simulink model "RLFactoryEnforceCrash6Opponents"  (R2020a)
settings: Solver=VariableStepAuto  StartTime=0.0  StopTime=60  RelTol=1e-3
undefined symbols (not defined in the file): BLOCKEDTIMER, EPS, getRandomSafeCoord, GoalRange, MAXVELOA, MAXVELOB, MAXVELOC, MAXVELOD, MAXVELOE, MAXVELOF, rl, RLStartX, RLStartY, SAFETYDISTANCEA, SAFETYDISTANCEB, SAFETYDISTANCEC, SAFETYDISTANCED, SAFETYDISTANCEE, SAFETYDISTANCEF, THRESHOLDA, THRESHOLDB, THRESHOLDC, THRESHOLDD, THRESHOLDE, THRESHOLDF, TSA, TSB, TSC, TSD, TSE, TSF, TSRL
libraries: rllib x1
(part 1 of 3)
settings Model: Creator=julius  LastModifiedBy=julius

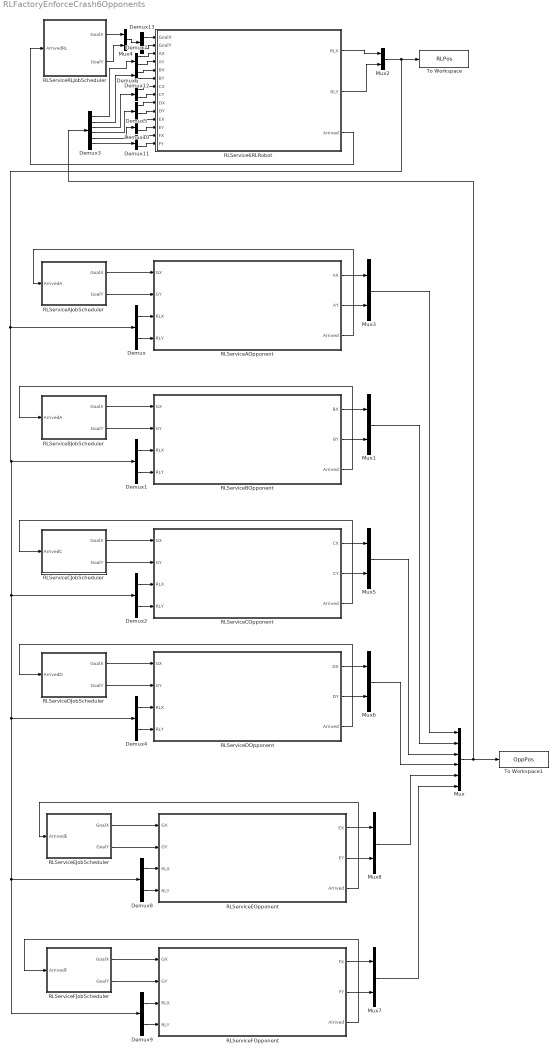
== system RLFactoryEnforceCrash6Opponents ==
  Demux{,1..2,4..13} (13 alike) : Demux  Outputs=2
  Demux3 : Demux  Outputs=6
  Mux : Mux  Inputs=6
  Mux{1..8} (8 alike) : Mux  Inputs=2
  RLService6RLRobot : Subsystem
  RLServiceAJobScheduler : Subsystem
  RLServiceAOpponent : Subsystem
  RLServiceBJobScheduler : Subsystem
  RLServiceBOpponent : Subsystem
  RLServiceCJobScheduler : Subsystem
  RLServiceCOpponent : Subsystem
  RLServiceDJobScheduler : Subsystem
  RLServiceDOpponent : Subsystem
  RLServiceEJobScheduler : Subsystem
  RLServiceEOpponent : Subsystem
  RLServiceFJobScheduler : Subsystem
  RLServiceFOpponent : Subsystem
  RLServiceRLJobScheduler : Subsystem
  To Workspace : ToWorkspace  VariableName=RLPos  SampleTime=TSRL
  To Workspace1 : ToWorkspace  VariableName=OppPos  SampleTime=TSRL
  wires:
  RLServiceAJobScheduler/1(GoalX) -> RLServiceAOpponent/1(GX)
  RLServiceAJobScheduler/2(GoalY) -> RLServiceAOpponent/2(GY)
  RLServiceAOpponent/3(Arrived) -> RLServiceAJobScheduler/1(ArrivedA)
  Demux/1 -> RLServiceAOpponent/3(RLX)
  Demux/2 -> RLServiceAOpponent/4(RLY)
  RLServiceBJobScheduler/1(GoalX) -> RLServiceBOpponent/1(GX)
  RLServiceBJobScheduler/2(GoalY) -> RLServiceBOpponent/2(GY)
  Demux1/1 -> RLServiceBOpponent/3(RLX)
  Demux1/2 -> RLServiceBOpponent/4(RLY)
  RLServiceBOpponent/1(BX) -> Mux1/1
  RLServiceBOpponent/2(BY) -> Mux1/2
  RLServiceAOpponent/1(AX) -> Mux3/1
  RLServiceAOpponent/2(AY) -> Mux3/2
  RLServiceBOpponent/3(Arrived) -> RLServiceBJobScheduler/1(ArrivedA)
  RLServiceRLJobScheduler/2(GoalY) -> Mux4/2
  RLServiceRLJobScheduler/1(GoalX) -> Mux4/1
  Mux4/1 -> Demux13/1
  Mux3/1 -> Mux/1
  Mux1/1 -> Mux/2
  Mux/1 -> Demux3/1, To Workspace1/1
  Demux3/1 -> Demux7/1
  Demux3/2 -> Demux12/1
  Demux13/1 -> RLService6RLRobot/1(GoalX)
  Demux13/2 -> RLService6RLRobot/2(GoalY)
  Demux7/1 -> RLService6RLRobot/3(AX)
  Demux7/2 -> RLService6RLRobot/4(AY)
  Demux12/1 -> RLService6RLRobot/5(BX)
  Demux12/2 -> RLService6RLRobot/6(BY)
  RLService6RLRobot/3(Arrived) -> RLServiceRLJobScheduler/1(ArrivedRL)
  RLService6RLRobot/1(RLX) -> Mux2/1
  RLService6RLRobot/2(RLY) -> Mux2/2
  RLServiceCJobScheduler/2(GoalY) -> RLServiceCOpponent/2(GY)
  Demux2/2 -> RLServiceCOpponent/4(RLY)
  RLServiceCOpponent/2(CY) -> Mux5/2
  RLServiceCJobScheduler/1(GoalX) -> RLServiceCOpponent/1(GX)
  RLServiceCOpponent/3(Arrived) -> RLServiceCJobScheduler/1(ArrivedC)
  RLServiceCOpponent/1(CX) -> Mux5/1
  Demux2/1 -> RLServiceCOpponent/3(RLX)
  RLServiceDJobScheduler/2(GoalY) -> RLServiceDOpponent/2(GY)
  Demux4/2 -> RLServiceDOpponent/4(RLY)
  RLServiceDOpponent/2(DY) -> Mux6/2
  RLServiceDJobScheduler/1(GoalX) -> RLServiceDOpponent/1(GX)
  RLServiceDOpponent/3(Arrived) -> RLServiceDJobScheduler/1(ArrivedD)
  RLServiceDOpponent/1(DX) -> Mux6/1
  Demux4/1 -> RLServiceDOpponent/3(RLX)
  Mux5/1 -> Mux/3
  Mux6/1 -> Mux/4
  Demux6/2 -> RLService6RLRobot/8(CY)
  Demux3/3 -> Demux6/1
  Demux6/1 -> RLService6RLRobot/7(CX)
  Demux8/2 -> RLServiceEOpponent/4(RLY)
  RLServiceEOpponent/1(EX) -> Mux8/1
  RLServiceEJobScheduler/1(GoalX) -> RLServiceEOpponent/1(GX)
  RLServiceEOpponent/2(EY) -> Mux8/2
  Mux8/1 -> Mux/5
  Demux8/1 -> RLServiceEOpponent/3(RLX)
  Demux9/2 -> RLServiceFOpponent/4(RLY)
  RLServiceFOpponent/3(Arrived) -> RLServiceFJobScheduler/1(ArrivedF)
  RLServiceEOpponent/3(Arrived) -> RLServiceEJobScheduler/1(ArrivedE)
  RLServiceFOpponent/1(FX) -> Mux7/1
  RLServiceEJobScheduler/2(GoalY) -> RLServiceEOpponent/2(GY)
  RLServiceFJobScheduler/1(GoalX) -> RLServiceFOpponent/1(GX)
  Mux2/1 -> Demux8/1, Demux9/1, Demux4/1, Demux2/1, Demux1/1, Demux/1, To Workspace/1
  RLServiceFOpponent/2(FY) -> Mux7/2
  Mux7/1 -> Mux/6
  RLServiceFJobScheduler/2(GoalY) -> RLServiceFOpponent/2(GY)
  Demux9/1 -> RLServiceFOpponent/3(RLX)
  Demux5/1 -> RLService6RLRobot/9(DX)
  Demux5/2 -> RLService6RLRobot/10(DY)
  Demux3/4 -> Demux5/1
  Demux10/1 -> RLService6RLRobot/11(EX)
  Demux10/2 -> RLService6RLRobot/12(EY)
  Demux11/1 -> RLService6RLRobot/13(FX)
  Demux11/2 -> RLService6RLRobot/14(FY)
  Demux3/5 -> Demux10/1
  Demux3/6 -> Demux11/1

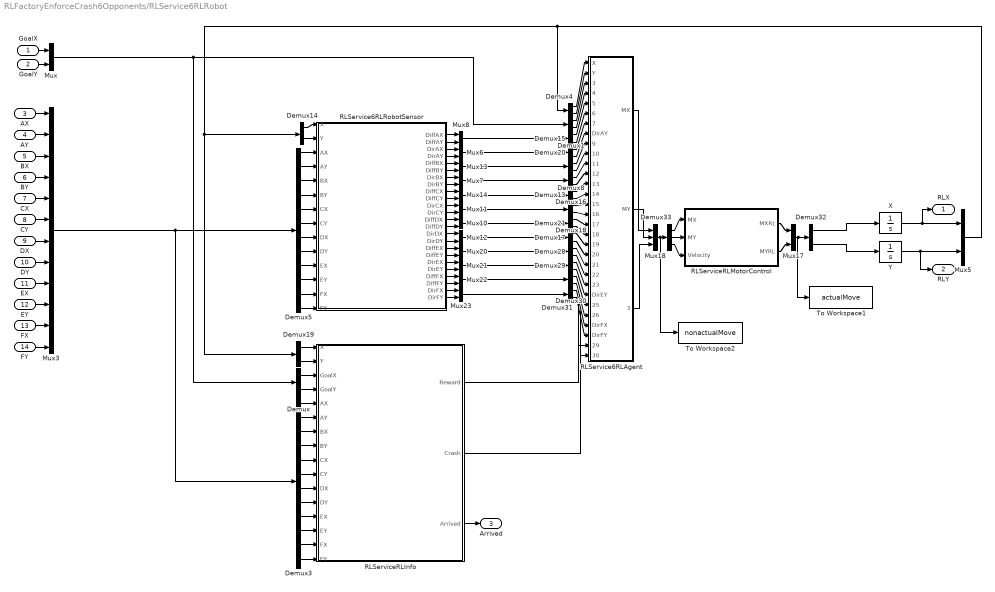
== system RLFactoryEnforceCrash6Opponents/RLService6RLRobot ==
  GoalX : Inport
  GoalY : Inport  Port=2
  AX : Inport  Port=3
  AY : Inport  Port=4
  BX : Inport  Port=5
  BY : Inport  Port=6
  CX : Inport  Port=7
  CY : Inport  Port=8
  DX : Inport  Port=9
  DY : Inport  Port=10
  EX : Inport  Port=11
  EY : Inport  Port=12
  FX : Inport  Port=13
  FY : Inport  Port=14
  Demux{,1,4,8,13..21,28..32} (18 alike) : Demux  Outputs=2
  Demux3 : Demux  Outputs=12
  Demux33 : Demux  Outputs=3
  Demux5 : Demux  Outputs=12
  Mux{,5..8,10..14,17,20..23} (15 alike) : Mux  Inputs=2
  Mux18 : Mux  Inputs=3
  Mux3 : Mux  Inputs=12
  RLService6RLAgent : Subsystem
  RLService6RLRobotSensor : Subsystem
  RLServiceRLInfo : Subsystem
  RLServiceRLMotorControl : Subsystem
  To Workspace1 : ToWorkspace  VariableName=actualMove  SampleTime=-1
  To Workspace2 : ToWorkspace  VariableName=nonactualMove  SampleTime=-1
  X : Integrator  InitialCondition=RLStartX
  Y : Integrator  InitialCondition=RLStartY
  RLX : Outport
  RLY : Outport  Port=2
  Arrived : Outport  Port=3
  wires:
  AX/1 -> Mux3/1
  X/1 -> Mux5/1, RLX/1
  Mux13/1 -> Demux8/1
  Demux19/1 -> RLServiceRLInfo/1(X)
  Demux4/1 -> RLService6RLAgent/1(X)
  Demux4/2 -> RLService6RLAgent/2(Y)
  Demux15/1 -> RLService6RLAgent/5(DiffAX)
  GoalX/1 -> Mux/1
  Demux20/2 -> RLService6RLAgent/8(DirAY)
  Demux19/2 -> RLServiceRLInfo/2(Y)
  Demux1/2 -> RLService6RLAgent/4(GoalY)
  Demux16/1 -> RLService6RLAgent/11(DirBX)
  Demux15/2 -> RLService6RLAgent/6(DiffAY)
  Demux/2 -> RLServiceRLInfo/4(GoalY)
  Demux1/1 -> RLService6RLAgent/3(GoalX)
  Y/1 -> RLY/1, Mux5/2
  RLService6RLAgent/2(MY) -> Mux18/2
  Mux3/1 -> Demux5/1, Demux3/1
  Demux20/1 -> RLService6RLAgent/7(DirAX)
  Demux8/1 -> RLService6RLAgent/9(DiffBX)
  BY/1 -> Mux3/4
  GoalY/1 -> Mux/2
  Mux5/1 -> Demux14/1, Demux19/1, Demux4/1
  Mux6/1 -> Demux20/1
  Demux/1 -> RLServiceRLInfo/3(GoalX)
  RLService6RLAgent/1(MX) -> Mux18/1
  Mux7/1 -> Demux16/1
  BX/1 -> Mux3/3
  Demux16/2 -> RLService6RLAgent/12(DirBY)
  AY/1 -> Mux3/2
  Demux8/2 -> RLService6RLAgent/10(DiffBY)
  Mux8/1 -> Demux15/1
  RLService6RLAgent/3(Velocity) -> Mux18/3
  CX/1 -> Mux3/5
  CY/1 -> Mux3/6
  DX/1 -> Mux3/7
  DY/1 -> Mux3/8
  Demux13/1 -> RLService6RLAgent/13(DiffCX)
  Demux18/2 -> RLService6RLAgent/16(DirCY)
  Demux13/2 -> RLService6RLAgent/14(DiffCY)
  Demux21/2 -> RLService6RLAgent/18(DiffDY)
  Demux17/1 -> RLService6RLAgent/19(DirDX)
  Demux17/2 -> RLService6RLAgent/20(DirDY)
  Demux18/1 -> RLService6RLAgent/15(DirCX)
  Demux21/1 -> RLService6RLAgent/17(DiffDX)
  Mux14/1 -> Demux13/1
  Mux11/1 -> Demux18/1
  Mux10/1 -> Demux21/1
  Mux12/1 -> Demux17/1
  FX/1 -> Mux3/11
  EY/1 -> Mux3/10
  EX/1 -> Mux3/9
  FY/1 -> Mux3/12
  Demux14/1 -> RLService6RLRobotSensor/1(X)
  Demux14/2 -> RLService6RLRobotSensor/2(Y)
  RLService6RLRobotSensor/1(DiffAX) -> Mux8/1
  RLService6RLRobotSensor/2(DiffAY) -> Mux8/2
  Mux/1 -> Demux1/1, Demux/1
  RLService6RLRobotSensor/3(DirAX) -> Mux6/1
  RLService6RLRobotSensor/4(DirAY) -> Mux6/2
  RLService6RLRobotSensor/5(DiffBX) -> Mux13/1
  RLService6RLRobotSensor/6(DiffBY) -> Mux13/2
  RLService6RLRobotSensor/7(DirBX) -> Mux7/1
  RLService6RLRobotSensor/8(DirBY) -> Mux7/2
  RLService6RLRobotSensor/9(DiffCX) -> Mux14/1
  RLService6RLRobotSensor/10(DiffCY) -> Mux14/2
  RLService6RLRobotSensor/11(DirCX) -> Mux11/1
  RLService6RLRobotSensor/12(DirCY) -> Mux11/2
  RLService6RLRobotSensor/13(DiffDX) -> Mux10/1
  RLService6RLRobotSensor/14(DiffDY) -> Mux10/2
  RLService6RLRobotSensor/15(DirDX) -> Mux12/1
  RLService6RLRobotSensor/16(DirDY) -> Mux12/2
  RLService6RLRobotSensor/17(DiffEX) -> Mux20/1
  RLService6RLRobotSensor/18(DiffEY) -> Mux20/2
  Demux28/1 -> RLService6RLAgent/21(DiffEX)
  Demux28/2 -> RLService6RLAgent/22(DiffEY)
  Mux20/1 -> Demux28/1
  Demux29/2 -> RLService6RLAgent/24(DirEY)
  Demux29/1 -> RLService6RLAgent/23(DirEX)
  RLService6RLRobotSensor/19(DirEX) -> Mux21/1
  RLService6RLRobotSensor/20(DirEY) -> Mux21/2
  Mux21/1 -> Demux29/1
  RLService6RLRobotSensor/21(DiffFX) -> Mux22/1
  RLService6RLRobotSensor/22(DiffFY) -> Mux22/2
  Demux30/1 -> RLService6RLAgent/25(DiffFX)
  Demux30/2 -> RLService6RLAgent/26(DiffFY)
  Mux22/1 -> Demux30/1
  RLService6RLRobotSensor/23(DirFX) -> Mux23/1
  RLService6RLRobotSensor/24(DirFY) -> Mux23/2
  Mux23/1 -> Demux31/1
  Demux31/1 -> RLService6RLAgent/27(DirFX)
  Demux31/2 -> RLService6RLAgent/28(DirFY)
  RLServiceRLMotorControl/1(MXRL) -> Mux17/1
  RLServiceRLMotorControl/2(MYRL) -> Mux17/2
  Mux17/1 -> To Workspace1/1, Demux32/1
  Demux32/1 -> X/1
  Demux32/2 -> Y/1
  Demux33/1 -> RLServiceRLMotorControl/1(MX)
  Demux33/2 -> RLServiceRLMotorControl/2(MY)
  Demux33/3 -> RLServiceRLMotorControl/3(Velocity)
  Mux18/1 -> Demux33/1, To Workspace2/1
  RLServiceRLInfo/3(Arrived) -> Arrived/1
  Demux3/1 -> RLServiceRLInfo/5(AX)
  Demux3/2 -> RLServiceRLInfo/6(AY)
  Demux3/3 -> RLServiceRLInfo/7(BX)
  Demux3/4 -> RLServiceRLInfo/8(BY)
  Demux3/5 -> RLServiceRLInfo/9(CX)
  Demux3/6 -> RLServiceRLInfo/10(CY)
  Demux3/7 -> RLServiceRLInfo/11(DX)
  Demux3/8 -> RLServiceRLInfo/12(DY)
  Demux3/9 -> RLServiceRLInfo/13(EX)
  Demux3/10 -> RLServiceRLInfo/14(EY)
  Demux3/11 -> RLServiceRLInfo/15(FX)
  Demux3/12 -> RLServiceRLInfo/16(FY)
  RLServiceRLInfo/1(Reward) -> RLService6RLAgent/29(Reward)
  RLServiceRLInfo/2(Crash) -> RLService6RLAgent/30(IsDone)
  Demux5/2 -> RLService6RLRobotSensor/4(AY)
  Demux5/3 -> RLService6RLRobotSensor/5(BX)
  Demux5/4 -> RLService6RLRobotSensor/6(BY)
  Demux5/5 -> RLService6RLRobotSensor/7(CX)
  Demux5/6 -> RLService6RLRobotSensor/8(CY)
  Demux5/7 -> RLService6RLRobotSensor/9(DX)
  Demux5/8 -> RLService6RLRobotSensor/10(DY)
  Demux5/9 -> RLService6RLRobotSensor/11(EX)
  Demux5/10 -> RLService6RLRobotSensor/12(EY)
  Demux5/11 -> RLService6RLRobotSensor/13(FX)
  Demux5/12 -> RLService6RLRobotSensor/14(FY)
  Demux5/1 -> RLService6RLRobotSensor/3(AX)

== system RLFactoryEnforceCrash6Opponents/RLServiceAJobScheduler ==
  ArrivedA : Inport
  Constant1 : Constant  Value=[[randi([-GoalRange,GoalRange],1),randi([-GoalRange,GoalRange],1)];[randi([-GoalRange,GoalRange],1),randi([-GoalRange,GoalRange],1)]]
  JobScheduler2 : MATLABSystem  System=JobScheduler  SimulateUsing=Interpreted execution
      mask Type: JobScheduler
      mask Display:
      | disp('JobScheduler');
      | port_label('input',1,'workstations');
      | port_label('input',2,'done');
      | port_label('output',1,'currentGoalX');
      | port_label('output',2,'currentGoalY');
  GoalX : Outport
  GoalY : Outport  Port=2
  wires:
  Constant1/1 -> JobScheduler2/1
  JobScheduler2/2 -> GoalY/1
  ArrivedA/1 -> JobScheduler2/2
  JobScheduler2/1 -> GoalX/1

== system RLFactoryEnforceCrash6Opponents/RLServiceAOpponent ==
  GX : Inport
  GY : Inport  Port=2
  RLX : Inport  Port=3
  RLY : Inport  Port=4
  Constant1 : Constant  Value=MAXVELOA
  Constant2 : Constant  Value=TSA
  Constant3 : Constant  Value=THRESHOLDA
  Demux : Demux  Outputs=6
  Demux1 : Demux  Outputs=2
  Demux11 : Demux  Outputs=3
  Demux2 : Demux  Outputs=2
  Mux : Mux  Inputs=2
  Mux2 : Mux  Inputs=3
  Mux9 : Mux  Inputs=6
  RLServiceAOpponentController : Subsystem
  X : Integrator  InitialCondition=getRandomSafeCoord(RLStartX,SAFETYDISTANCEA,EPS)
  Y : Integrator  InitialCondition=getRandomSafeCoord(RLStartY,SAFETYDISTANCEA,EPS)
  ZOA : ZeroOrderHold  SampleTime=TSA
  AX : Outport
  AY : Outport  Port=2
  Arrived : Outport  Port=3
  wires:
  RLServiceAOpponentController/1(Arrived) -> Arrived/1
  Demux/4 -> RLServiceAOpponentController/4(GoalY)
  Demux/6 -> RLServiceAOpponentController/6(RLY)
  X/1 -> Mux/1
  RLY/1 -> Mux9/6
  Demux/5 -> RLServiceAOpponentController/5(RLX)
  GY/1 -> Mux9/4
  Demux/1 -> RLServiceAOpponentController/1(X)
  Y/1 -> Mux/2
  Mux/1 -> Demux1/1, Demux2/1
  Mux9/1 -> ZOA/1
  Demux/3 -> RLServiceAOpponentController/3(GoalX)
  Demux/2 -> RLServiceAOpponentController/2(Y)
  RLX/1 -> Mux9/5
  ZOA/1 -> Demux/1
  GX/1 -> Mux9/3
  Mux2/1 -> Demux11/1
  Demux1/1 -> Mux9/1
  Demux1/2 -> Mux9/2
  Constant2/1 -> Mux2/2
  Constant1/1 -> Mux2/1
  Constant3/1 -> Mux2/3
  Demux2/1 -> AX/1
  Demux2/2 -> AY/1
  RLServiceAOpponentController/3(MY) -> Y/1
  RLServiceAOpponentController/2(MX) -> X/1
  Demux11/1 -> RLServiceAOpponentController/7(MaxVelo)
  Demux11/2 -> RLServiceAOpponentController/8(TS)
  Demux11/3 -> RLServiceAOpponentController/9(THRESHOLD)

== system RLFactoryEnforceCrash6Opponents/RLServiceBJobScheduler ==
  ArrivedA : Inport
  Constant1 : Constant  Value=[[randi([-GoalRange,GoalRange],1),randi([-GoalRange,GoalRange],1)];[randi([-GoalRange,GoalRange],1),randi([-GoalRange,GoalRange],1)]]
  JobScheduler2 : MATLABSystem  System=JobScheduler  SimulateUsing=Interpreted execution
      mask Type: JobScheduler
      mask Display:
      | disp('JobScheduler');
      | port_label('input',1,'workstations');
      | port_label('input',2,'done');
      | port_label('output',1,'currentGoalX');
      | port_label('output',2,'currentGoalY');
  GoalX : Outport
  GoalY : Outport  Port=2
  wires:
  Constant1/1 -> JobScheduler2/1
  JobScheduler2/2 -> GoalY/1
  ArrivedA/1 -> JobScheduler2/2
  JobScheduler2/1 -> GoalX/1

== system RLFactoryEnforceCrash6Opponents/RLServiceBOpponent ==
  GX : Inport
  GY : Inport  Port=2
  RLX : Inport  Port=3
  RLY : Inport  Port=4
  Constant1 : Constant  Value=MAXVELOB
  Constant2 : Constant  Value=TSB
  Constant3 : Constant  Value=THRESHOLDB
  Demux : Demux  Outputs=6
  Demux1 : Demux  Outputs=2
  Demux11 : Demux  Outputs=3
  Demux2 : Demux  Outputs=2
  Mux : Mux  Inputs=2
  Mux2 : Mux  Inputs=3
  Mux9 : Mux  Inputs=6
  RLServiceAOpponentController : Subsystem
  X : Integrator  InitialCondition=getRandomSafeCoord(RLStartX,SAFETYDISTANCEB,EPS)
  Y : Integrator  InitialCondition=getRandomSafeCoord(RLStartY,SAFETYDISTANCEB,EPS)
  ZOB : ZeroOrderHold  SampleTime=TSB
  BX : Outport
  BY : Outport  Port=2
  Arrived : Outport  Port=3
  wires:
  RLServiceAOpponentController/3(MY) -> Y/1
  RLX/1 -> Mux9/5
  Demux11/1 -> RLServiceAOpponentController/7(MaxVelo)
  Constant2/1 -> Mux2/2
  RLServiceAOpponentController/2(MX) -> X/1
  Mux9/1 -> ZOB/1
  Constant3/1 -> Mux2/3
  Demux1/2 -> Mux9/2
  Demux/1 -> RLServiceAOpponentController/1(X)
  GY/1 -> Mux9/4
  Demux/4 -> RLServiceAOpponentController/4(GoalY)
  RLServiceAOpponentController/1(Arrived) -> Arrived/1
  X/1 -> Mux/1
  Mux/1 -> Demux1/1, Demux2/1
  Demux/6 -> RLServiceAOpponentController/6(RLY)
  Demux/3 -> RLServiceAOpponentController/3(GoalX)
  Demux1/1 -> Mux9/1
  Demux11/2 -> RLServiceAOpponentController/8(TS)
  Demux2/1 -> BX/1
  RLY/1 -> Mux9/6
  Demux/2 -> RLServiceAOpponentController/2(Y)
  Demux11/3 -> RLServiceAOpponentController/9(THRESHOLD)
  ZOB/1 -> Demux/1
  Demux2/2 -> BY/1
  Mux2/1 -> Demux11/1
  Constant1/1 -> Mux2/1
  GX/1 -> Mux9/3
  Y/1 -> Mux/2
  Demux/5 -> RLServiceAOpponentController/5(RLX)

== system RLFactoryEnforceCrash6Opponents/RLServiceCJobScheduler ==
  ArrivedC : Inport
  Constant1 : Constant  Value=[[randi([-5,5],1),randi([-5,5],1)];[randi([-5,5],1),randi([-5,5],1)]]
  JobScheduler2 : MATLABSystem  System=JobScheduler  SimulateUsing=Interpreted execution
      mask Type: JobScheduler
      mask Display:
      | disp('JobScheduler');
      | port_label('input',1,'workstations');
      | port_label('input',2,'done');
      | port_label('output',1,'currentGoalX');
      | port_label('output',2,'currentGoalY');
  GoalX : Outport
  GoalY : Outport  Port=2
  wires:
  Constant1/1 -> JobScheduler2/1
  JobScheduler2/2 -> GoalY/1
  ArrivedC/1 -> JobScheduler2/2
  JobScheduler2/1 -> GoalX/1

== system RLFactoryEnforceCrash6Opponents/RLServiceCOpponent ==
  GX : Inport
  GY : Inport  Port=2
  RLX : Inport  Port=3
  RLY : Inport  Port=4
  Constant1 : Constant  Value=MAXVELOC
  Constant2 : Constant  Value=TSC
  Constant3 : Constant  Value=THRESHOLDC
  Demux : Demux  Outputs=6
  Demux1 : Demux  Outputs=2
  Demux11 : Demux  Outputs=3
  Demux2 : Demux  Outputs=2
  Mux : Mux  Inputs=2
  Mux2 : Mux  Inputs=3
  Mux9 : Mux  Inputs=6
  RLServiceAOpponentController : Subsystem
  X : Integrator  InitialCondition=getRandomSafeCoord(RLStartX,SAFETYDISTANCEC,EPS)
  Y : Integrator  InitialCondition=getRandomSafeCoord(RLStartY,SAFETYDISTANCEC,EPS)
  ZOC : ZeroOrderHold  SampleTime=TSC
  CX : Outport
  CY : Outport  Port=2
  Arrived : Outport  Port=3
  wires:
  RLServiceAOpponentController/3(MY) -> Y/1
  RLX/1 -> Mux9/5
  Demux11/1 -> RLServiceAOpponentController/7(MaxVelo)
  Constant2/1 -> Mux2/2
  RLServiceAOpponentController/2(MX) -> X/1
  Mux9/1 -> ZOC/1
  Constant3/1 -> Mux2/3
  Demux1/2 -> Mux9/2
  Demux/1 -> RLServiceAOpponentController/1(X)
  GY/1 -> Mux9/4
  Demux/4 -> RLServiceAOpponentController/4(GoalY)
  RLServiceAOpponentController/1(Arrived) -> Arrived/1
  X/1 -> Mux/1
  Mux/1 -> Demux1/1, Demux2/1
  Demux/6 -> RLServiceAOpponentController/6(RLY)
  Demux/3 -> RLServiceAOpponentController/3(GoalX)
  Demux1/1 -> Mux9/1
  Demux11/2 -> RLServiceAOpponentController/8(TS)
  Demux2/1 -> CX/1
  RLY/1 -> Mux9/6
  Demux/2 -> RLServiceAOpponentController/2(Y)
  Demux11/3 -> RLServiceAOpponentController/9(THRESHOLD)
  ZOC/1 -> Demux/1
  Demux2/2 -> CY/1
  Mux2/1 -> Demux11/1
  Constant1/1 -> Mux2/1
  GX/1 -> Mux9/3
  Y/1 -> Mux/2
  Demux/5 -> RLServiceAOpponentController/5(RLX)

== system RLFactoryEnforceCrash6Opponents/RLServiceDJobScheduler ==
  ArrivedD : Inport
  Constant1 : Constant  Value=[[randi([-GoalRange,GoalRange],1),randi([-GoalRange,GoalRange],1)];[randi([-GoalRange,GoalRange],1),randi([-GoalRange,GoalRange],1)]]
  JobScheduler2 : MATLABSystem  System=JobScheduler  SimulateUsing=Interpreted execution
      mask Type: JobScheduler
      mask Display:
      | disp('JobScheduler');
      | port_label('input',1,'workstations');
      | port_label('input',2,'done');
      | port_label('output',1,'currentGoalX');
      | port_label('output',2,'currentGoalY');
  GoalX : Outport
  GoalY : Outport  Port=2
  wires:
  Constant1/1 -> JobScheduler2/1
  JobScheduler2/2 -> GoalY/1
  ArrivedD/1 -> JobScheduler2/2
  JobScheduler2/1 -> GoalX/1

== system RLFactoryEnforceCrash6Opponents/RLServiceDOpponent ==
  GX : Inport
  GY : Inport  Port=2
  RLX : Inport  Port=3
  RLY : Inport  Port=4
  Constant1 : Constant  Value=MAXVELOD
  Constant2 : Constant  Value=TSD
  Constant3 : Constant  Value=THRESHOLDD
  Demux : Demux  Outputs=6
  Demux1 : Demux  Outputs=2
  Demux11 : Demux  Outputs=3
  Demux2 : Demux  Outputs=2
  Mux : Mux  Inputs=2
  Mux2 : Mux  Inputs=3
  Mux9 : Mux  Inputs=6
  RLServiceAOpponentController : Subsystem
  X : Integrator  InitialCondition=getRandomSafeCoord(RLStartX,SAFETYDISTANCED,EPS)
  Y : Integrator  InitialCondition=getRandomSafeCoord(RLStartY,SAFETYDISTANCED,EPS)
  ZOB : ZeroOrderHold  SampleTime=TSD
  DX : Outport
  DY : Outport  Port=2
  Arrived : Outport  Port=3
  wires:
  RLServiceAOpponentController/3(MY) -> Y/1
  RLX/1 -> Mux9/5
  Demux11/1 -> RLServiceAOpponentController/7(MaxVelo)
  Constant2/1 -> Mux2/2
  RLServiceAOpponentController/2(MX) -> X/1
  Mux9/1 -> ZOB/1
  Constant3/1 -> Mux2/3
  Demux1/2 -> Mux9/2
  Demux/1 -> RLServiceAOpponentController/1(X)
  GY/1 -> Mux9/4
  Demux/4 -> RLServiceAOpponentController/4(GoalY)
  RLServiceAOpponentController/1(Arrived) -> Arrived/1
  X/1 -> Mux/1
  Mux/1 -> Demux1/1, Demux2/1
  Demux/6 -> RLServiceAOpponentController/6(RLY)
  Demux/3 -> RLServiceAOpponentController/3(GoalX)
  Demux1/1 -> Mux9/1
  Demux11/2 -> RLServiceAOpponentController/8(TS)
  Demux2/1 -> DX/1
  RLY/1 -> Mux9/6
  Demux/2 -> RLServiceAOpponentController/2(Y)
  Demux11/3 -> RLServiceAOpponentController/9(THRESHOLD)
  ZOB/1 -> Demux/1
  Demux2/2 -> DY/1
  Mux2/1 -> Demux11/1
  Constant1/1 -> Mux2/1
  GX/1 -> Mux9/3
  Y/1 -> Mux/2
  Demux/5 -> RLServiceAOpponentController/5(RLX)

== system RLFactoryEnforceCrash6Opponents/RLServiceEJobScheduler ==
  ArrivedE : Inport
  Constant1 : Constant  Value=[[randi([-GoalRange,GoalRange],1),randi([-GoalRange,GoalRange],1)];[randi([-GoalRange,GoalRange],1),randi([-GoalRange,GoalRange],1)]]
  JobScheduler2 : MATLABSystem  System=JobScheduler  SimulateUsing=Interpreted execution
      mask Type: JobScheduler
      mask Display:
      | disp('JobScheduler');
      | port_label('input',1,'workstations');
      | port_label('input',2,'done');
      | port_label('output',1,'currentGoalX');
      | port_label('output',2,'currentGoalY');
  GoalX : Outport
  GoalY : Outport  Port=2
  wires:
  Constant1/1 -> JobScheduler2/1
  JobScheduler2/2 -> GoalY/1
  ArrivedE/1 -> JobScheduler2/2
  JobScheduler2/1 -> GoalX/1

== system RLFactoryEnforceCrash6Opponents/RLServiceEOpponent ==
  GX : Inport
  GY : Inport  Port=2
  RLX : Inport  Port=3
  RLY : Inport  Port=4
  Constant1 : Constant  Value=MAXVELOE
  Constant2 : Constant  Value=TSE
  Constant3 : Constant  Value=THRESHOLDE
  Demux : Demux  Outputs=6
  Demux1 : Demux  Outputs=2
  Demux11 : Demux  Outputs=3
  Demux2 : Demux  Outputs=2
  Mux : Mux  Inputs=2
  Mux2 : Mux  Inputs=3
  Mux9 : Mux  Inputs=6
  RLServiceAOpponentController : Subsystem
  X : Integrator  InitialCondition=getRandomSafeCoord(RLStartX,SAFETYDISTANCEE, EPS)
  Y : Integrator  InitialCondition=getRandomSafeCoord(RLStartY,SAFETYDISTANCEE, EPS)
  ZOE : ZeroOrderHold  SampleTime=TSE
  EX : Outport
  EY : Outport  Port=2
  Arrived : Outport  Port=3
  wires:
  RLServiceAOpponentController/1(Arrived) -> Arrived/1
  Demux/4 -> RLServiceAOpponentController/4(GoalY)
  Demux/6 -> RLServiceAOpponentController/6(RLY)
  X/1 -> Mux/1
  RLY/1 -> Mux9/6
  Demux/5 -> RLServiceAOpponentController/5(RLX)
  GY/1 -> Mux9/4
  Demux/1 -> RLServiceAOpponentController/1(X)
  Y/1 -> Mux/2
  Mux/1 -> Demux1/1, Demux2/1
  Mux9/1 -> ZOE/1
  Demux/3 -> RLServiceAOpponentController/3(GoalX)
  Demux/2 -> RLServiceAOpponentController/2(Y)
  RLX/1 -> Mux9/5
  ZOE/1 -> Demux/1
  GX/1 -> Mux9/3
  Mux2/1 -> Demux11/1
  Demux1/1 -> Mux9/1
  Demux1/2 -> Mux9/2
  Constant2/1 -> Mux2/2
  Constant1/1 -> Mux2/1
  Constant3/1 -> Mux2/3
  Demux2/1 -> EX/1
  Demux2/2 -> EY/1
  RLServiceAOpponentController/3(MY) -> Y/1
  RLServiceAOpponentController/2(MX) -> X/1
  Demux11/1 -> RLServiceAOpponentController/7(MaxVelo)
  Demux11/2 -> RLServiceAOpponentController/8(TS)
  Demux11/3 -> RLServiceAOpponentController/9(THRESHOLD)

== system RLFactoryEnforceCrash6Opponents/RLServiceFJobScheduler ==
  ArrivedF : Inport
  Constant1 : Constant  Value=[[randi([-GoalRange,GoalRange],1),randi([-GoalRange,GoalRange],1)];[randi([-GoalRange,GoalRange],1),randi([-GoalRange,GoalRange],1)]]
  JobScheduler2 : MATLABSystem  System=JobScheduler  SimulateUsing=Interpreted execution
      mask Type: JobScheduler
      mask Display:
      | disp('JobScheduler');
      | port_label('input',1,'workstations');
      | port_label('input',2,'done');
      | port_label('output',1,'currentGoalX');
      | port_label('output',2,'currentGoalY');
  GoalX : Outport
  GoalY : Outport  Port=2
  wires:
  Constant1/1 -> JobScheduler2/1
  JobScheduler2/2 -> GoalY/1
  ArrivedF/1 -> JobScheduler2/2
  JobScheduler2/1 -> GoalX/1

== system RLFactoryEnforceCrash6Opponents/RLServiceFOpponent ==
  GX : Inport
  GY : Inport  Port=2
  RLX : Inport  Port=3
  RLY : Inport  Port=4
  Constant1 : Constant  Value=MAXVELOF
  Constant2 : Constant  Value=TSF
  Constant3 : Constant  Value=THRESHOLDF
  Demux : Demux  Outputs=6
  Demux1 : Demux  Outputs=2
  Demux11 : Demux  Outputs=3
  Demux2 : Demux  Outputs=2
  Mux : Mux  Inputs=2
  Mux2 : Mux  Inputs=3
  Mux9 : Mux  Inputs=6
  RLServiceAOpponentController : Subsystem
  X : Integrator  InitialCondition=getRandomSafeCoord(RLStartX,SAFETYDISTANCEF,EPS)
  Y : Integrator  InitialCondition=getRandomSafeCoord(RLStartY,SAFETYDISTANCEF,EPS)
  ZOF : ZeroOrderHold  SampleTime=TSF
  FX : Outport
  FY : Outport  Port=2
  Arrived : Outport  Port=3
  wires:
  RLServiceAOpponentController/3(MY) -> Y/1
  RLX/1 -> Mux9/5
  Demux11/1 -> RLServiceAOpponentController/7(MaxVelo)
  Constant2/1 -> Mux2/2
  RLServiceAOpponentController/2(MX) -> X/1
  Mux9/1 -> ZOF/1
  Constant3/1 -> Mux2/3
  Demux1/2 -> Mux9/2
  Demux/1 -> RLServiceAOpponentController/1(X)
  GY/1 -> Mux9/4
  Demux/4 -> RLServiceAOpponentController/4(GoalY)
  RLServiceAOpponentController/1(Arrived) -> Arrived/1
  X/1 -> Mux/1
  Mux/1 -> Demux1/1, Demux2/1
  Demux/6 -> RLServiceAOpponentController/6(RLY)
  Demux/3 -> RLServiceAOpponentController/3(GoalX)
  Demux1/1 -> Mux9/1
  Demux11/2 -> RLServiceAOpponentController/8(TS)
  Demux2/1 -> FX/1
  RLY/1 -> Mux9/6
  Demux/2 -> RLServiceAOpponentController/2(Y)
  Demux11/3 -> RLServiceAOpponentController/9(THRESHOLD)
  ZOF/1 -> Demux/1
  Demux2/2 -> FY/1
  Mux2/1 -> Demux11/1
  Constant1/1 -> Mux2/1
  GX/1 -> Mux9/3
  Y/1 -> Mux/2
  Demux/5 -> RLServiceAOpponentController/5(RLX)

== system RLFactoryEnforceCrash6Opponents/RLServiceRLJobScheduler ==
  note: Goal for RL Robot is 100,100. Realistically, this goal is unimportant as the RL agent acts randomly.
  ArrivedRL : Inport
  Constant : Constant  Value=[5,5]
  JobScheduler1 : MATLABSystem  System=JobScheduler  SimulateUsing=Code generation
      mask Type: JobScheduler
      mask Display:
      | disp('JobScheduler');
      | port_label('input',1,'workstations');
      | port_label('input',2,'done');
      | port_label('output',1,'currentGoalX');
      | port_label('output',2,'currentGoalY');
  Mux2 : Mux  Inputs=2
  To Workspace2 : ToWorkspace  VariableName=Job  SampleTime=0.25
  GoalX : Outport
  GoalY : Outport  Port=2
  wires:
  Constant/1 -> JobScheduler1/1
  JobScheduler1/2 -> Mux2/2, GoalY/1
  ArrivedRL/1 -> JobScheduler1/2
  JobScheduler1/1 -> Mux2/1, GoalX/1
  Mux2/1 -> To Workspace2/1

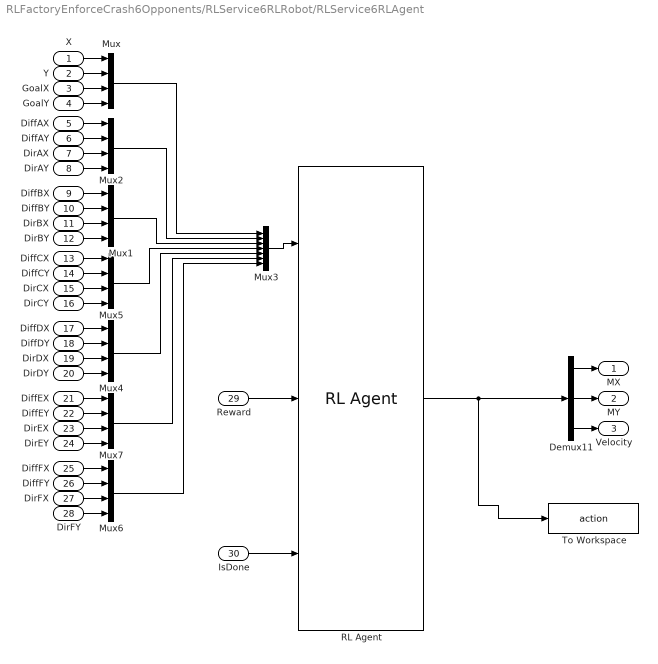
== system RLFactoryEnforceCrash6Opponents/RLService6RLRobot/RLService6RLAgent ==
  X : Inport
  Y : Inport  Port=2
  GoalX : Inport  Port=3
  GoalY : Inport  Port=4
  DiffAX : Inport  Port=5
  DiffAY : Inport  Port=6
  DirAX : Inport  Port=7
  DirAY : Inport  Port=8
  DiffBX : Inport  Port=9
  DiffBY : Inport  Port=10
  DirBX : Inport  Port=11
  DirBY : Inport  Port=12
  DiffCX : Inport  Port=13
  DiffCY : Inport  Port=14
  DirCX : Inport  Port=15
  DirCY : Inport  Port=16
  DiffDX : Inport  Port=17
  DiffDY : Inport  Port=18
  DirDX : Inport  Port=19
  DirDY : Inport  Port=20
  DiffEX : Inport  Port=21
  DiffEY : Inport  Port=22
  DirEX : Inport  Port=23
  DirEY : Inport  Port=24
  DiffFX : Inport  Port=25
  DiffFY : Inport  Port=26
  DirFX : Inport  Port=27
  DirFY : Inport  Port=28
  Reward : Inport  Port=29
  IsDone : Inport  Port=30
  Demux11 : Demux  Outputs=3
  Mux{,1..2,4..7} (7 alike) : Mux
  Mux3 : Mux  Inputs=7
  RL Agent : rllib/RL Agent  Agent=rl.util.PolicyInstance.get()  ProvideReward=on  ProvideIsDone=on  ProvideCumRwd=off  TreatAsDirectFeedthrough=on  CollectLoggedSignals=on  CollectModelStates=on
  To Workspace : ToWorkspace  VariableName=action  SampleTime=TSRL
  MX : Outport
  MY : Outport  Port=2
  Velocity : Outport  Port=3
  wires:
  IsDone/1 -> RL Agent/3
  Demux11/1 -> MX/1
  Reward/1 -> RL Agent/2
  DirAX/1 -> Mux2/3
  GoalY/1 -> Mux/4
  DiffAX/1 -> Mux2/1
  X/1 -> Mux/1
  GoalX/1 -> Mux/3
  DirAY/1 -> Mux2/4
  DiffAY/1 -> Mux2/2
  Y/1 -> Mux/2
  DiffBX/1 -> Mux1/1
  DiffBY/1 -> Mux1/2
  DirBX/1 -> Mux1/3
  DirBY/1 -> Mux1/4
  Mux2/1 -> Mux3/2
  Mux3/1 -> RL Agent/1
  Mux/1 -> Mux3/1
  Mux1/1 -> Mux3/3
  Demux11/2 -> MY/1
  Demux11/3 -> Velocity/1
  DiffDY/1 -> Mux4/2
  Mux5/1 -> Mux3/4
  DiffCY/1 -> Mux5/2
  DirDY/1 -> Mux4/4
  DirCX/1 -> Mux5/3
  DiffDX/1 -> Mux4/1
  Mux4/1 -> Mux3/5
  DiffCX/1 -> Mux5/1
  DirCY/1 -> Mux5/4
  DirDX/1 -> Mux4/3
  DirFY/1 -> Mux6/4
  DiffFX/1 -> Mux6/1
  DiffEX/1 -> Mux7/1
  DiffEY/1 -> Mux7/2
  DiffFY/1 -> Mux6/2
  DirFX/1 -> Mux6/3
  DirEY/1 -> Mux7/4
  DirEX/1 -> Mux7/3
  Mux7/1 -> Mux3/6
  Mux6/1 -> Mux3/7
  RL Agent/1 -> To Workspace/1, Demux11/1

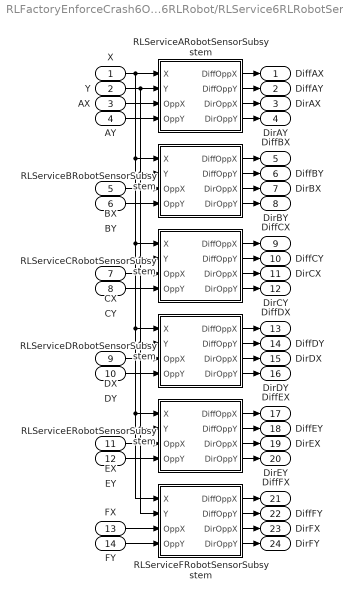
== system RLFactoryEnforceCrash6Opponents/RLService6RLRobot/RLService6RLRobotSensor ==
  X : Inport
  Y : Inport  Port=2
  AX : Inport  Port=3
  AY : Inport  Port=4
  BX : Inport  Port=5
  BY : Inport  Port=6
  CX : Inport  Port=7
  CY : Inport  Port=8
  DX : Inport  Port=9
  DY : Inport  Port=10
  EX : Inport  Port=11
  EY : Inport  Port=12
  FX : Inport  Port=13
  FY : Inport  Port=14
  RLServiceARobotSensorSubsystem : Subsystem
  RLServiceBRobotSensorSubsystem : Subsystem
  RLServiceCRobotSensorSubsystem : Subsystem
  RLServiceDRobotSensorSubsystem : Subsystem
  RLServiceERobotSensorSubsystem : Subsystem
  RLServiceFRobotSensorSubsystem : Subsystem
  DiffAX : Outport
  DiffAY : Outport  Port=2
  DirAX : Outport  Port=3
  DirAY : Outport  Port=4
  DiffBX : Outport  Port=5
  DiffBY : Outport  Port=6
  DirBX : Outport  Port=7
  DirBY : Outport  Port=8
  DiffCX : Outport  Port=9
  DiffCY : Outport  Port=10
  DirCX : Outport  Port=11
  DirCY : Outport  Port=12
  DiffDX : Outport  Port=13
  DiffDY : Outport  Port=14
  DirDX : Outport  Port=15
  DirDY : Outport  Port=16
  DiffEX : Outport  Port=17
  DiffEY : Outport  Port=18
  DirEX : Outport  Port=19
  DirEY : Outport  Port=20
  DiffFX : Outport  Port=21
  DiffFY : Outport  Port=22
  DirFX : Outport  Port=23
  DirFY : Outport  Port=24
  wires:
  RLServiceBRobotSensorSubsystem/3(DirOppX) -> DirBX/1
  BY/1 -> RLServiceBRobotSensorSubsystem/4(OppY)
  BX/1 -> RLServiceBRobotSensorSubsystem/3(OppX)
  RLServiceARobotSensorSubsystem/4(DirOppY) -> DirAY/1
  RLServiceBRobotSensorSubsystem/4(DirOppY) -> DirBY/1
  RLServiceBRobotSensorSubsystem/2(DiffOppY) -> DiffBY/1
  RLServiceARobotSensorSubsystem/3(DirOppX) -> DirAX/1
  RLServiceBRobotSensorSubsystem/1(DiffOppX) -> DiffBX/1
  AX/1 -> RLServiceARobotSensorSubsystem/3(OppX)
  AY/1 -> RLServiceARobotSensorSubsystem/4(OppY)
  RLServiceARobotSensorSubsystem/1(DiffOppX) -> DiffAX/1
  RLServiceARobotSensorSubsystem/2(DiffOppY) -> DiffAY/1
  RLServiceCRobotSensorSubsystem/1(DiffOppX) -> DiffCX/1
  CX/1 -> RLServiceCRobotSensorSubsystem/3(OppX)
  RLServiceCRobotSensorSubsystem/2(DiffOppY) -> DiffCY/1
  RLServiceCRobotSensorSubsystem/4(DirOppY) -> DirCY/1
  CY/1 -> RLServiceCRobotSensorSubsystem/4(OppY)
  RLServiceCRobotSensorSubsystem/3(DirOppX) -> DirCX/1
  RLServiceDRobotSensorSubsystem/3(DirOppX) -> DirDX/1
  DY/1 -> RLServiceDRobotSensorSubsystem/4(OppY)
  RLServiceDRobotSensorSubsystem/4(DirOppY) -> DirDY/1
  RLServiceDRobotSensorSubsystem/2(DiffOppY) -> DiffDY/1
  DX/1 -> RLServiceDRobotSensorSubsystem/3(OppX)
  RLServiceDRobotSensorSubsystem/1(DiffOppX) -> DiffDX/1
  RLServiceFRobotSensorSubsystem/1(DiffOppX) -> DiffFX/1
  RLServiceERobotSensorSubsystem/3(DirOppX) -> DirEX/1
  RLServiceFRobotSensorSubsystem/3(DirOppX) -> DirFX/1
  RLServiceERobotSensorSubsystem/2(DiffOppY) -> DiffEY/1
  RLServiceERobotSensorSubsystem/4(DirOppY) -> DirEY/1
  RLServiceERobotSensorSubsystem/1(DiffOppX) -> DiffEX/1
  FY/1 -> RLServiceFRobotSensorSubsystem/4(OppY)
  EY/1 -> RLServiceERobotSensorSubsystem/4(OppY)
  RLServiceFRobotSensorSubsystem/4(DirOppY) -> DirFY/1
  RLServiceFRobotSensorSubsystem/2(DiffOppY) -> DiffFY/1
  EX/1 -> RLServiceERobotSensorSubsystem/3(OppX)
  FX/1 -> RLServiceFRobotSensorSubsystem/3(OppX)
  X/1 -> RLServiceFRobotSensorSubsystem/1(X), RLServiceERobotSensorSubsystem/1(X), RLServiceDRobotSensorSubsystem/1(X), RLServiceCRobotSensorSubsystem/1(X), RLServiceBRobotSensorSubsystem/1(X), RLServiceARobotSensorSubsystem/1(X)
  Y/1 -> RLServiceCRobotSensorSubsystem/2(Y), RLServiceFRobotSensorSubsystem/2(Y), RLServiceERobotSensorSubsystem/2(Y), RLServiceDRobotSensorSubsystem/2(Y), RLServiceBRobotSensorSubsystem/2(Y), RLServiceARobotSensorSubsystem/2(Y)

== system RLFactoryEnforceCrash6Opponents/RLService6RLRobot/RLServiceRLInfo ==
  X : Inport
  Y : Inport  Port=2
  GoalX : Inport  Port=3
  GoalY : Inport  Port=4
  AX : Inport  Port=5
  AY : Inport  Port=6
  BX : Inport  Port=7
  BY : Inport  Port=8
  CX : Inport  Port=9
  CY : Inport  Port=10
  DX : Inport  Port=11
  DY : Inport  Port=12
  EX : Inport  Port=13
  EY : Inport  Port=14
  FX : Inport  Port=15
  FY : Inport  Port=16
  RLServiceCrashDetector : Subsystem
  RLServiceGoalTracker : Subsystem
  RLServiceReward : Subsystem
  To Workspace1 : ToWorkspace  VariableName=Crash  SampleTime=0.25
  Reward : Outport
  Crash : Outport  Port=2
  Arrived : Outport  Port=3
  wires:
  BY/1 -> RLServiceCrashDetector/6(BY)
  GoalY/1 -> RLServiceGoalTracker/4(GoalY)
  AX/1 -> RLServiceCrashDetector/3(AX)
  RLServiceGoalTracker/2(Arrived) -> Arrived/1, RLServiceReward/2(Arrived)
  Y/1 -> RLServiceGoalTracker/2(Y), RLServiceCrashDetector/2(Y)
  GoalX/1 -> RLServiceGoalTracker/3(GoalX)
  BX/1 -> RLServiceCrashDetector/5(BX)
  RLServiceReward/1(Reward) -> Reward/1
  AY/1 -> RLServiceCrashDetector/4(AY)
  X/1 -> RLServiceGoalTracker/1(X), RLServiceCrashDetector/1(X)
  RLServiceGoalTracker/1(Dist) -> RLServiceReward/1(DistGoal)
  RLServiceCrashDetector/2(Crash) -> RLServiceReward/3(Crash), Crash/1, To Workspace1/1
  RLServiceCrashDetector/1(BelowThreshold) -> RLServiceReward/4(BelowThreshold)
  CX/1 -> RLServiceCrashDetector/7(CX)
  CY/1 -> RLServiceCrashDetector/8(CY)
  DX/1 -> RLServiceCrashDetector/9(DX)
  DY/1 -> RLServiceCrashDetector/10(DY)
  EX/1 -> RLServiceCrashDetector/11(EX)
  EY/1 -> RLServiceCrashDetector/12(EY)
  FX/1 -> RLServiceCrashDetector/13(FX)
  FY/1 -> RLServiceCrashDetector/14(FY)

== system RLFactoryEnforceCrash6Opponents/RLService6RLRobot/RLServiceRLMotorControl ==
  MX : Inport
  MY : Inport  Port=2
  Velocity : Inport  Port=3
  RLServiceRLAdjustVelocity : Subsystem
  MXRL : Outport
  MYRL : Outport  Port=2
  wires:
  RLServiceRLAdjustVelocity/1(AdjMX) -> MXRL/1
  RLServiceRLAdjustVelocity/2(AdjMY) -> MYRL/1
  MX/1 -> RLServiceRLAdjustVelocity/1(MoveX)
  MY/1 -> RLServiceRLAdjustVelocity/2(MoveY)
  Velocity/1 -> RLServiceRLAdjustVelocity/3(Velocity)

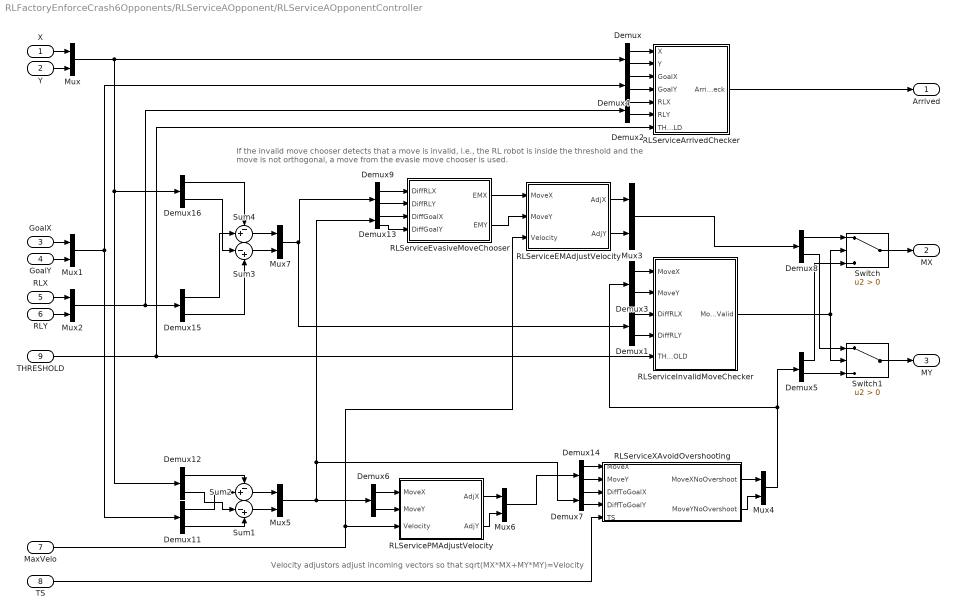
== system RLFactoryEnforceCrash6Opponents/RLServiceAOpponent/RLServiceAOpponentController ==
  note: If the invalid move chooser detects that a move is invalid, i.e.,
      | the RL robot is inside the threshold and the move is not orthogonal, a move from the evasie move chooser is used.
  note: Velocity adjustors adjust incoming vectors so that sqrt(MX*MX+MY*MY)=Velocity
  X : Inport
  Y : Inport  Port=2
  GoalX : Inport  Port=3
  GoalY : Inport  Port=4
  RLX : Inport  Port=5
  RLY : Inport  Port=6
  MaxVelo : Inport  Port=7
  TS : Inport  Port=8
  THRESHOLD : Inport  Port=9
  Demux{,1..9,11..16} (16 alike) : Demux  Outputs=2
  Mux{,1..7} (8 alike) : Mux  Inputs=2
  RLServiceArrivedChecker : Subsystem
  RLServiceEMAdjustVelocity : Subsystem
  RLServiceEvasiveMoveChooser : Subsystem
  RLServiceInvalidMoveChecker : Subsystem
  RLServicePMAdjustVelocity : Subsystem
  RLServiceXAvoidOvershooting : Subsystem
  Sum1 : Sum  Inputs=|-+
  Sum2 : Sum  Inputs=-+|
  Sum3 : Sum  Inputs=|-+
  Sum4 : Sum  Inputs=-+|
  Switch : Switch  Criteria=u2 > Threshold
  Switch1 : Switch  Criteria=u2 > Threshold
  Arrived : Outport
  MX : Outport  Port=2
  MY : Outport  Port=3
  wires:
  GoalX/1 -> Mux1/1
  GoalY/1 -> Mux1/2
  RLServiceArrivedChecker/1(ArrivedCheck) -> Arrived/1
  Demux/1 -> RLServiceArrivedChecker/1(X)
  Demux/2 -> RLServiceArrivedChecker/2(Y)
  Demux4/1 -> RLServiceArrivedChecker/3(GoalX)
  Demux4/2 -> RLServiceArrivedChecker/4(GoalY)
  X/1 -> Mux/1
  Y/1 -> Mux/2
  RLX/1 -> Mux2/1
  RLY/1 -> Mux2/2
  Demux3/1 -> RLServiceInvalidMoveChecker/1(MoveX)
  Demux8/1 -> Switch/1
  Demux5/2 -> Switch1/3
  Demux8/2 -> Switch1/1
  THRESHOLD/1 -> RLServiceArrivedChecker/7(THRESHOLD), RLServiceInvalidMoveChecker/5(THRESHOLD)
  Demux3/2 -> RLServiceInvalidMoveChecker/2(MoveY)
  Demux5/1 -> Switch/3
  RLServiceInvalidMoveChecker/1(MoveInValid) -> Switch/2, Switch1/2
  Switch/1 -> MX/1
  Switch1/1 -> MY/1
  Mux5/1 -> Demux6/1, Demux7/1, Demux13/1
  Demux6/2 -> RLServicePMAdjustVelocity/2(MoveY)
  Mux1/1 -> Demux4/1, Demux11/1
  TS/1 -> RLServiceXAvoidOvershooting/5(TS)
  MaxVelo/1 -> RLServiceEMAdjustVelocity/3(Velocity), RLServicePMAdjustVelocity/3(Velocity)
  RLServicePMAdjustVelocity/1(AdjX) -> Mux6/1
  RLServicePMAdjustVelocity/2(AdjY) -> Mux6/2
  RLServiceEvasiveMoveChooser/1(EMX) -> RLServiceEMAdjustVelocity/1(MoveX)
  RLServiceEvasiveMoveChooser/2(EMY) -> RLServiceEMAdjustVelocity/2(MoveY)
  RLServiceEMAdjustVelocity/1(AdjX) -> Mux3/1
  RLServiceEMAdjustVelocity/2(AdjY) -> Mux3/2
  Mux3/1 -> Demux8/1
  RLServiceXAvoidOvershooting/1(MoveXNoOvershoot) -> Mux4/1
  RLServiceXAvoidOvershooting/2(MoveYNoOvershoot) -> Mux4/2
  Mux4/1 -> Demux5/1, Demux3/1
  Sum2/1 -> Mux5/1
  Sum1/1 -> Mux5/2
  Demux6/1 -> RLServicePMAdjustVelocity/1(MoveX)
  Demux7/1 -> RLServiceXAvoidOvershooting/3(DiffToGoalX)
  Demux7/2 -> RLServiceXAvoidOvershooting/4(DiffToGoalY)
  Demux13/1 -> RLServiceEvasiveMoveChooser/3(DiffGoalX)
  Demux13/2 -> RLServiceEvasiveMoveChooser/4(DiffGoalY)
  Demux11/1 -> Sum2/2
  Demux12/2 -> Sum1/1
  Demux11/2 -> Sum1/2
  Demux12/1 -> Sum2/1
  Demux14/1 -> RLServiceXAvoidOvershooting/1(MoveX)
  Demux14/2 -> RLServiceXAvoidOvershooting/2(MoveY)
  Mux6/1 -> Demux14/1
  Sum3/1 -> Mux7/2
  Demux16/1 -> Sum4/1
  Sum4/1 -> Mux7/1
  Mux/1 -> Demux12/1, Demux16/1, Demux/1
  Mux2/1 -> Demux2/1, Demux15/1
  Demux15/2 -> Sum3/2
  Demux15/1 -> Sum4/2
  Demux16/2 -> Sum3/1
  Demux9/1 -> RLServiceEvasiveMoveChooser/1(DiffRLX)
  Demux9/2 -> RLServiceEvasiveMoveChooser/2(DiffRLY)
  Mux7/1 -> Demux1/1, Demux9/1
  Demux1/1 -> RLServiceInvalidMoveChecker/3(DiffRLX)
  Demux1/2 -> RLServiceInvalidMoveChecker/4(DiffRLY)
  Demux2/2 -> RLServiceArrivedChecker/6(RLY)
  Demux2/1 -> RLServiceArrivedChecker/5(RLX)

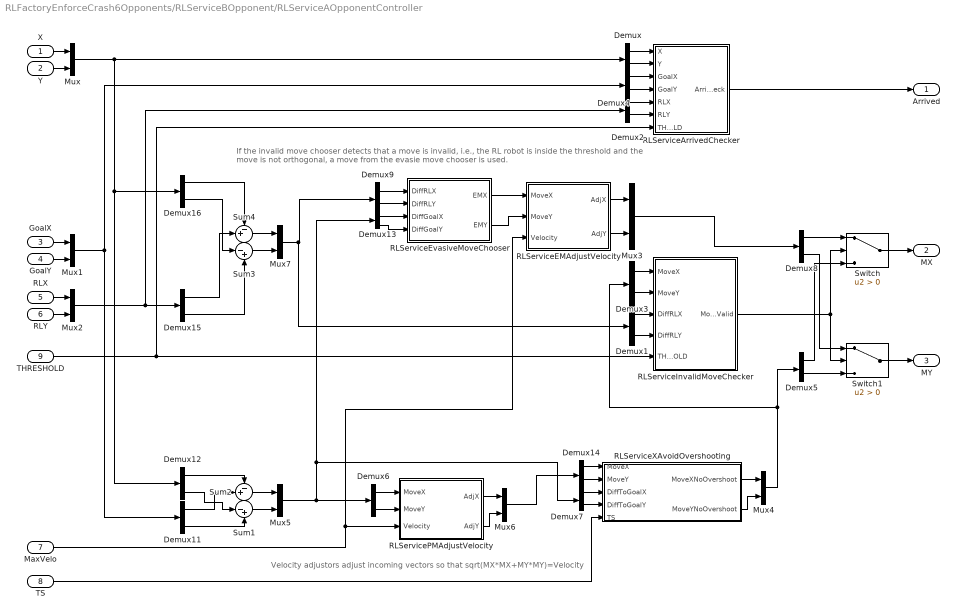
== system RLFactoryEnforceCrash6Opponents/RLServiceBOpponent/RLServiceAOpponentController ==
  note: If the invalid move chooser detects that a move is invalid, i.e.,
      | the RL robot is inside the threshold and the move is not orthogonal, a move from the evasie move chooser is used.
  note: Velocity adjustors adjust incoming vectors so that sqrt(MX*MX+MY*MY)=Velocity
  X : Inport
  Y : Inport  Port=2
  GoalX : Inport  Port=3
  GoalY : Inport  Port=4
  RLX : Inport  Port=5
  RLY : Inport  Port=6
  MaxVelo : Inport  Port=7
  TS : Inport  Port=8
  THRESHOLD : Inport  Port=9
  Demux{,1..9,11..16} (16 alike) : Demux  Outputs=2
  Mux{,1..7} (8 alike) : Mux  Inputs=2
  RLServiceArrivedChecker : Subsystem
  RLServiceEMAdjustVelocity : Subsystem
  RLServiceEvasiveMoveChooser : Subsystem
  RLServiceInvalidMoveChecker : Subsystem
  RLServicePMAdjustVelocity : Subsystem
  RLServiceXAvoidOvershooting : Subsystem
  Sum1 : Sum  Inputs=|-+
  Sum2 : Sum  Inputs=-+|
  Sum3 : Sum  Inputs=|-+
  Sum4 : Sum  Inputs=-+|
  Switch : Switch  Criteria=u2 > Threshold
  Switch1 : Switch  Criteria=u2 > Threshold
  Arrived : Outport
  MX : Outport  Port=2
  MY : Outport  Port=3
  wires:
  GoalX/1 -> Mux1/1
  GoalY/1 -> Mux1/2
  RLServiceArrivedChecker/1(ArrivedCheck) -> Arrived/1
  Demux/1 -> RLServiceArrivedChecker/1(X)
  Demux/2 -> RLServiceArrivedChecker/2(Y)
  Demux4/1 -> RLServiceArrivedChecker/3(GoalX)
  Demux4/2 -> RLServiceArrivedChecker/4(GoalY)
  X/1 -> Mux/1
  Y/1 -> Mux/2
  RLX/1 -> Mux2/1
  RLY/1 -> Mux2/2
  Demux3/1 -> RLServiceInvalidMoveChecker/1(MoveX)
  Demux8/1 -> Switch/1
  Demux5/2 -> Switch1/3
  Demux8/2 -> Switch1/1
  THRESHOLD/1 -> RLServiceArrivedChecker/7(THRESHOLD), RLServiceInvalidMoveChecker/5(THRESHOLD)
  Demux3/2 -> RLServiceInvalidMoveChecker/2(MoveY)
  Demux5/1 -> Switch/3
  RLServiceInvalidMoveChecker/1(MoveInValid) -> Switch/2, Switch1/2
  Switch/1 -> MX/1
  Switch1/1 -> MY/1
  Mux5/1 -> Demux6/1, Demux7/1, Demux13/1
  Demux6/2 -> RLServicePMAdjustVelocity/2(MoveY)
  Mux1/1 -> Demux4/1, Demux11/1
  TS/1 -> RLServiceXAvoidOvershooting/5(TS)
  MaxVelo/1 -> RLServiceEMAdjustVelocity/3(Velocity), RLServicePMAdjustVelocity/3(Velocity)
  RLServicePMAdjustVelocity/1(AdjX) -> Mux6/1
  RLServicePMAdjustVelocity/2(AdjY) -> Mux6/2
  RLServiceEvasiveMoveChooser/1(EMX) -> RLServiceEMAdjustVelocity/1(MoveX)
  RLServiceEvasiveMoveChooser/2(EMY) -> RLServiceEMAdjustVelocity/2(MoveY)
  RLServiceEMAdjustVelocity/1(AdjX) -> Mux3/1
  RLServiceEMAdjustVelocity/2(AdjY) -> Mux3/2
  Mux3/1 -> Demux8/1
  RLServiceXAvoidOvershooting/1(MoveXNoOvershoot) -> Mux4/1
  RLServiceXAvoidOvershooting/2(MoveYNoOvershoot) -> Mux4/2
  Mux4/1 -> Demux5/1, Demux3/1
  Sum2/1 -> Mux5/1
  Sum1/1 -> Mux5/2
  Demux6/1 -> RLServicePMAdjustVelocity/1(MoveX)
  Demux7/1 -> RLServiceXAvoidOvershooting/3(DiffToGoalX)
  Demux7/2 -> RLServiceXAvoidOvershooting/4(DiffToGoalY)
  Demux13/1 -> RLServiceEvasiveMoveChooser/3(DiffGoalX)
  Demux13/2 -> RLServiceEvasiveMoveChooser/4(DiffGoalY)
  Demux11/1 -> Sum2/2
  Demux12/2 -> Sum1/1
  Demux11/2 -> Sum1/2
  Demux12/1 -> Sum2/1
  Demux14/1 -> RLServiceXAvoidOvershooting/1(MoveX)
  Demux14/2 -> RLServiceXAvoidOvershooting/2(MoveY)
  Mux6/1 -> Demux14/1
  Sum3/1 -> Mux7/2
  Demux16/1 -> Sum4/1
  Sum4/1 -> Mux7/1
  Mux/1 -> Demux12/1, Demux16/1, Demux/1
  Mux2/1 -> Demux2/1, Demux15/1
  Demux15/2 -> Sum3/2
  Demux15/1 -> Sum4/2
  Demux16/2 -> Sum3/1
  Demux9/1 -> RLServiceEvasiveMoveChooser/1(DiffRLX)
  Demux9/2 -> RLServiceEvasiveMoveChooser/2(DiffRLY)
  Mux7/1 -> Demux1/1, Demux9/1
  Demux1/1 -> RLServiceInvalidMoveChecker/3(DiffRLX)
  Demux1/2 -> RLServiceInvalidMoveChecker/4(DiffRLY)
  Demux2/2 -> RLServiceArrivedChecker/6(RLY)
  Demux2/1 -> RLServiceArrivedChecker/5(RLX)

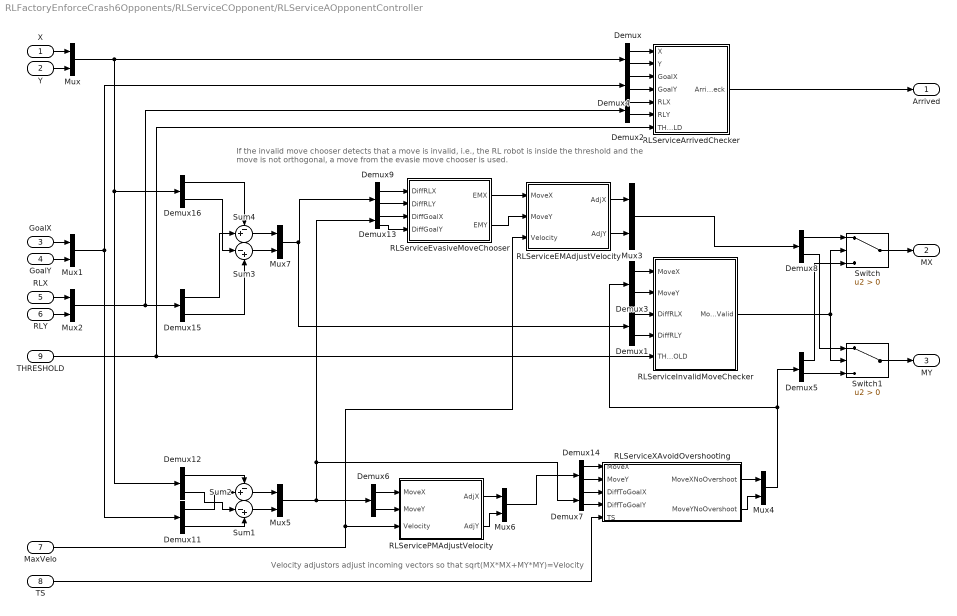
== system RLFactoryEnforceCrash6Opponents/RLServiceCOpponent/RLServiceAOpponentController ==
  note: If the invalid move chooser detects that a move is invalid, i.e.,
      | the RL robot is inside the threshold and the move is not orthogonal, a move from the evasie move chooser is used.
  note: Velocity adjustors adjust incoming vectors so that sqrt(MX*MX+MY*MY)=Velocity
  X : Inport
  Y : Inport  Port=2
  GoalX : Inport  Port=3
  GoalY : Inport  Port=4
  RLX : Inport  Port=5
  RLY : Inport  Port=6
  MaxVelo : Inport  Port=7
  TS : Inport  Port=8
  THRESHOLD : Inport  Port=9
  Demux{,1..9,11..16} (16 alike) : Demux  Outputs=2
  Mux{,1..7} (8 alike) : Mux  Inputs=2
  RLServiceArrivedChecker : Subsystem
  RLServiceEMAdjustVelocity : Subsystem
  RLServiceEvasiveMoveChooser : Subsystem
  RLServiceInvalidMoveChecker : Subsystem
  RLServicePMAdjustVelocity : Subsystem
  RLServiceXAvoidOvershooting : Subsystem
  Sum1 : Sum  Inputs=|-+
  Sum2 : Sum  Inputs=-+|
  Sum3 : Sum  Inputs=|-+
  Sum4 : Sum  Inputs=-+|
  Switch : Switch  Criteria=u2 > Threshold
  Switch1 : Switch  Criteria=u2 > Threshold
  Arrived : Outport
  MX : Outport  Port=2
  MY : Outport  Port=3
  wires:
  GoalX/1 -> Mux1/1
  GoalY/1 -> Mux1/2
  RLServiceArrivedChecker/1(ArrivedCheck) -> Arrived/1
  Demux/1 -> RLServiceArrivedChecker/1(X)
  Demux/2 -> RLServiceArrivedChecker/2(Y)
  Demux4/1 -> RLServiceArrivedChecker/3(GoalX)
  Demux4/2 -> RLServiceArrivedChecker/4(GoalY)
  X/1 -> Mux/1
  Y/1 -> Mux/2
  RLX/1 -> Mux2/1
  RLY/1 -> Mux2/2
  Demux3/1 -> RLServiceInvalidMoveChecker/1(MoveX)
  Demux8/1 -> Switch/1
  Demux5/2 -> Switch1/3
  Demux8/2 -> Switch1/1
  THRESHOLD/1 -> RLServiceArrivedChecker/7(THRESHOLD), RLServiceInvalidMoveChecker/5(THRESHOLD)
  Demux3/2 -> RLServiceInvalidMoveChecker/2(MoveY)
  Demux5/1 -> Switch/3
  RLServiceInvalidMoveChecker/1(MoveInValid) -> Switch/2, Switch1/2
  Switch/1 -> MX/1
  Switch1/1 -> MY/1
  Mux5/1 -> Demux6/1, Demux7/1, Demux13/1
  Demux6/2 -> RLServicePMAdjustVelocity/2(MoveY)
  Mux1/1 -> Demux4/1, Demux11/1
  TS/1 -> RLServiceXAvoidOvershooting/5(TS)
  MaxVelo/1 -> RLServiceEMAdjustVelocity/3(Velocity), RLServicePMAdjustVelocity/3(Velocity)
  RLServicePMAdjustVelocity/1(AdjX) -> Mux6/1
  RLServicePMAdjustVelocity/2(AdjY) -> Mux6/2
  RLServiceEvasiveMoveChooser/1(EMX) -> RLServiceEMAdjustVelocity/1(MoveX)
  RLServiceEvasiveMoveChooser/2(EMY) -> RLServiceEMAdjustVelocity/2(MoveY)
  RLServiceEMAdjustVelocity/1(AdjX) -> Mux3/1
  RLServiceEMAdjustVelocity/2(AdjY) -> Mux3/2
  Mux3/1 -> Demux8/1
  RLServiceXAvoidOvershooting/1(MoveXNoOvershoot) -> Mux4/1
  RLServiceXAvoidOvershooting/2(MoveYNoOvershoot) -> Mux4/2
  Mux4/1 -> Demux5/1, Demux3/1
  Sum2/1 -> Mux5/1
  Sum1/1 -> Mux5/2
  Demux6/1 -> RLServicePMAdjustVelocity/1(MoveX)
  Demux7/1 -> RLServiceXAvoidOvershooting/3(DiffToGoalX)
  Demux7/2 -> RLServiceXAvoidOvershooting/4(DiffToGoalY)
  Demux13/1 -> RLServiceEvasiveMoveChooser/3(DiffGoalX)
  Demux13/2 -> RLServiceEvasiveMoveChooser/4(DiffGoalY)
  Demux11/1 -> Sum2/2
  Demux12/2 -> Sum1/1
  Demux11/2 -> Sum1/2
  Demux12/1 -> Sum2/1
  Demux14/1 -> RLServiceXAvoidOvershooting/1(MoveX)
  Demux14/2 -> RLServiceXAvoidOvershooting/2(MoveY)
  Mux6/1 -> Demux14/1
  Sum3/1 -> Mux7/2
  Demux16/1 -> Sum4/1
  Sum4/1 -> Mux7/1
  Mux/1 -> Demux12/1, Demux16/1, Demux/1
  Mux2/1 -> Demux2/1, Demux15/1
  Demux15/2 -> Sum3/2
  Demux15/1 -> Sum4/2
  Demux16/2 -> Sum3/1
  Demux9/1 -> RLServiceEvasiveMoveChooser/1(DiffRLX)
  Demux9/2 -> RLServiceEvasiveMoveChooser/2(DiffRLY)
  Mux7/1 -> Demux1/1, Demux9/1
  Demux1/1 -> RLServiceInvalidMoveChecker/3(DiffRLX)
  Demux1/2 -> RLServiceInvalidMoveChecker/4(DiffRLY)
  Demux2/2 -> RLServiceArrivedChecker/6(RLY)
  Demux2/1 -> RLServiceArrivedChecker/5(RLX)

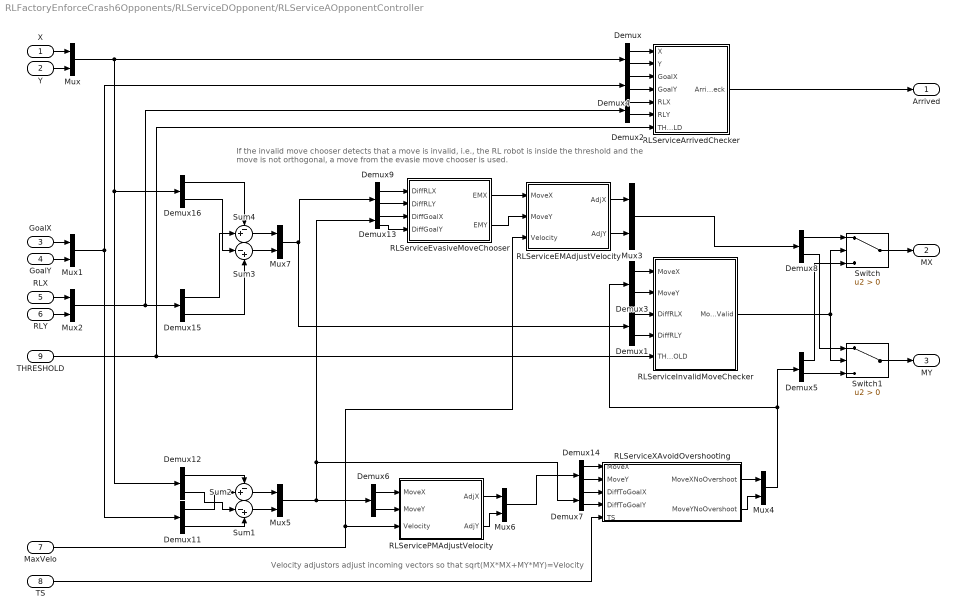
== system RLFactoryEnforceCrash6Opponents/RLServiceDOpponent/RLServiceAOpponentController ==
  note: If the invalid move chooser detects that a move is invalid, i.e.,
      | the RL robot is inside the threshold and the move is not orthogonal, a move from the evasie move chooser is used.
  note: Velocity adjustors adjust incoming vectors so that sqrt(MX*MX+MY*MY)=Velocity
  X : Inport
  Y : Inport  Port=2
  GoalX : Inport  Port=3
  GoalY : Inport  Port=4
  RLX : Inport  Port=5
  RLY : Inport  Port=6
  MaxVelo : Inport  Port=7
  TS : Inport  Port=8
  THRESHOLD : Inport  Port=9
  Demux{,1..9,11..16} (16 alike) : Demux  Outputs=2
  Mux{,1..7} (8 alike) : Mux  Inputs=2
  RLServiceArrivedChecker : Subsystem
  RLServiceEMAdjustVelocity : Subsystem
  RLServiceEvasiveMoveChooser : Subsystem
  RLServiceInvalidMoveChecker : Subsystem
  RLServicePMAdjustVelocity : Subsystem
  RLServiceXAvoidOvershooting : Subsystem
  Sum1 : Sum  Inputs=|-+
  Sum2 : Sum  Inputs=-+|
  Sum3 : Sum  Inputs=|-+
  Sum4 : Sum  Inputs=-+|
  Switch : Switch  Criteria=u2 > Threshold
  Switch1 : Switch  Criteria=u2 > Threshold
  Arrived : Outport
  MX : Outport  Port=2
  MY : Outport  Port=3
  wires:
  GoalX/1 -> Mux1/1
  GoalY/1 -> Mux1/2
  RLServiceArrivedChecker/1(ArrivedCheck) -> Arrived/1
  Demux/1 -> RLServiceArrivedChecker/1(X)
  Demux/2 -> RLServiceArrivedChecker/2(Y)
  Demux4/1 -> RLServiceArrivedChecker/3(GoalX)
  Demux4/2 -> RLServiceArrivedChecker/4(GoalY)
  X/1 -> Mux/1
  Y/1 -> Mux/2
  RLX/1 -> Mux2/1
  RLY/1 -> Mux2/2
  Demux3/1 -> RLServiceInvalidMoveChecker/1(MoveX)
  Demux8/1 -> Switch/1
  Demux5/2 -> Switch1/3
  Demux8/2 -> Switch1/1
  THRESHOLD/1 -> RLServiceArrivedChecker/7(THRESHOLD), RLServiceInvalidMoveChecker/5(THRESHOLD)
  Demux3/2 -> RLServiceInvalidMoveChecker/2(MoveY)
  Demux5/1 -> Switch/3
  RLServiceInvalidMoveChecker/1(MoveInValid) -> Switch/2, Switch1/2
  Switch/1 -> MX/1
  Switch1/1 -> MY/1
  Mux5/1 -> Demux6/1, Demux7/1, Demux13/1
  Demux6/2 -> RLServicePMAdjustVelocity/2(MoveY)
  Mux1/1 -> Demux4/1, Demux11/1
  TS/1 -> RLServiceXAvoidOvershooting/5(TS)
  MaxVelo/1 -> RLServiceEMAdjustVelocity/3(Velocity), RLServicePMAdjustVelocity/3(Velocity)
  RLServicePMAdjustVelocity/1(AdjX) -> Mux6/1
  RLServicePMAdjustVelocity/2(AdjY) -> Mux6/2
  RLServiceEvasiveMoveChooser/1(EMX) -> RLServiceEMAdjustVelocity/1(MoveX)
  RLServiceEvasiveMoveChooser/2(EMY) -> RLServiceEMAdjustVelocity/2(MoveY)
  RLServiceEMAdjustVelocity/1(AdjX) -> Mux3/1
  RLServiceEMAdjustVelocity/2(AdjY) -> Mux3/2
  Mux3/1 -> Demux8/1
  RLServiceXAvoidOvershooting/1(MoveXNoOvershoot) -> Mux4/1
  RLServiceXAvoidOvershooting/2(MoveYNoOvershoot) -> Mux4/2
  Mux4/1 -> Demux5/1, Demux3/1
  Sum2/1 -> Mux5/1
  Sum1/1 -> Mux5/2
  Demux6/1 -> RLServicePMAdjustVelocity/1(MoveX)
  Demux7/1 -> RLServiceXAvoidOvershooting/3(DiffToGoalX)
  Demux7/2 -> RLServiceXAvoidOvershooting/4(DiffToGoalY)
  Demux13/1 -> RLServiceEvasiveMoveChooser/3(DiffGoalX)
  Demux13/2 -> RLServiceEvasiveMoveChooser/4(DiffGoalY)
  Demux11/1 -> Sum2/2
  Demux12/2 -> Sum1/1
  Demux11/2 -> Sum1/2
  Demux12/1 -> Sum2/1
  Demux14/1 -> RLServiceXAvoidOvershooting/1(MoveX)
  Demux14/2 -> RLServiceXAvoidOvershooting/2(MoveY)
  Mux6/1 -> Demux14/1
  Sum3/1 -> Mux7/2
  Demux16/1 -> Sum4/1
  Sum4/1 -> Mux7/1
  Mux/1 -> Demux12/1, Demux16/1, Demux/1
  Mux2/1 -> Demux2/1, Demux15/1
  Demux15/2 -> Sum3/2
  Demux15/1 -> Sum4/2
  Demux16/2 -> Sum3/1
  Demux9/1 -> RLServiceEvasiveMoveChooser/1(DiffRLX)
  Demux9/2 -> RLServiceEvasiveMoveChooser/2(DiffRLY)
  Mux7/1 -> Demux1/1, Demux9/1
  Demux1/1 -> RLServiceInvalidMoveChecker/3(DiffRLX)
  Demux1/2 -> RLServiceInvalidMoveChecker/4(DiffRLY)
  Demux2/2 -> RLServiceArrivedChecker/6(RLY)
  Demux2/1 -> RLServiceArrivedChecker/5(RLX)
